simulink model "VIPLTrgtPosChk"  (R2018b)
settings: Solver=FixedStepDiscrete  StartTime=0.0  StopTime=10.0  FixedStep=0.01  RelTol=1e-3
undefined symbols (not defined in the file or in its folder): SecRwLtStBkReclnTrgtPos, SecRwLtStFwdBkwdTrgtPos, SecRwLtStLgrstInwdOtwdTrgtPos, SecRwLtStLgrstUpwdDnwdTrgtPos, SecRwLtStZeroTrgtPos, VIPL557TrgtPos_Set
settings Model: Creator=sn2xws  LastModifiedBy=sn2xws
settings Model: ModifiedHistory=|
  | 2024.7.1 V3.0.0 557模式流程V1.9
  | 2024.8.15 V3.0.1增加 avl=1反馈，avl=0时将目标位置设为最大
  | 2024.9.18 V3.0.2 智享6s，7s接口变更
  | 2024.11.15 V3.0.3 再无法计算出有效位置时，都给最小智享位置做为目标位置
settings DataIOCC: SaveFormat=StructureWithTime
settings OptimizationCC: DefaultParameterBehavior=Inlined  EnhancedBackFolding=on  PassReuseOutputArgsAs=Individual arguments  ZeroExternalMemoryAtStartup=off  ZeroInternalMemoryAtStartup=off  OptimizeBlockOrder=speed  DifferentSizesBufferReuse=on  OptimizationCustomize=off
settings DebuggingCC: ParameterTunabilityLossMsg=error
settings HardwareCC: ProdBitPerPointer=32  ProdBitPerSizeT=32  ProdBitPerPtrDiffT=32  ProdLargestAtomicFloat=None  ProdWordSize=32  ProdHWDeviceType=Renesas->RH850
settings SFSimCC: MATLABDynamicMemAlloc=off
settings SFSimCC: SimCustomHeaderCode=|
  | #include "qmath.h"
  | #include "MsminterfDet.h"
  | #include "wisenjoy.h"
settings SFSimCC: SimUserSources=|
  | qmath.c
  | MsminterfDet.c
  | wisenjoy.c
settings RTWCC: SystemTargetFile=autosar.tlc  GenCodeOnly=on  TemplateMakefile=ert_default_tmf  Description=AUTOSAR  GenerateReport=on  IncludeHyperlinkInReport=on  LaunchReport=on  GenerateTraceInfo=on  GenerateTraceReport=on  GenerateTraceReportSl=on  GenerateTraceReportSf=on  GenerateTraceReportEml=on
settings CodeAppCC: ForceParamTrailComments=on  IgnoreCustomStorageClasses=off  OperatorAnnotations=on  SimulinkDataObjDesc=on  SFDataObjDesc=on  InsertBlockDesc=on
settings STFCustomTargetCC: TargetLangStandard=C99 (ISO)  MultiwordLength=256  ParMdlRefBuildCompliant=on  CompOptLevelCompliant=on  IncludeMdlTerminateFcn=off  CombineOutputUpdateFcns=on  SuppressErrorStatus=on  ERTCustomFileBanners=on  SupportNonFinite=off  SupportComplex=off  SupportContinuousTime=off  SupportNonInlinedSFcns=off  RemoveResetFunc=on  MATLABClassNameForMDSCustomization=Simulink.SoftwareTarget.ERTCustomization  AutosarCompliant=on  UseToolchainInfoCompliant=on  LookupTableObjectStructAxisOrder=2,1,3,4,...  LUTObjectStructOrderEvenSpacing=Size,Table,Breakpoints  SystemTargetFile=autosar.tlc
settings ERTTargetCC: TargetLangStandard=C99 (ISO)  ConcurrentExecutionCompliant=off  IncludeMdlTerminateFcn=off  SuppressErrorStatus=on  SupportNonFinite=off  SupportComplex=off  ModelStepFunctionPrototypeControlCompliant=off  CPPClassGenCompliant=off  AutosarCompliant=on  LookupTableObjectStructAxisOrder=2,1,3,4,...  LUTObjectStructOrderEvenSpacing=Size,Table,Breakpoints  InlinedParameterPlacement=NonHierarchical  ERTCustomFileTemplate=example_file_process.tlc  ERTFilePackagingFormat=Compact

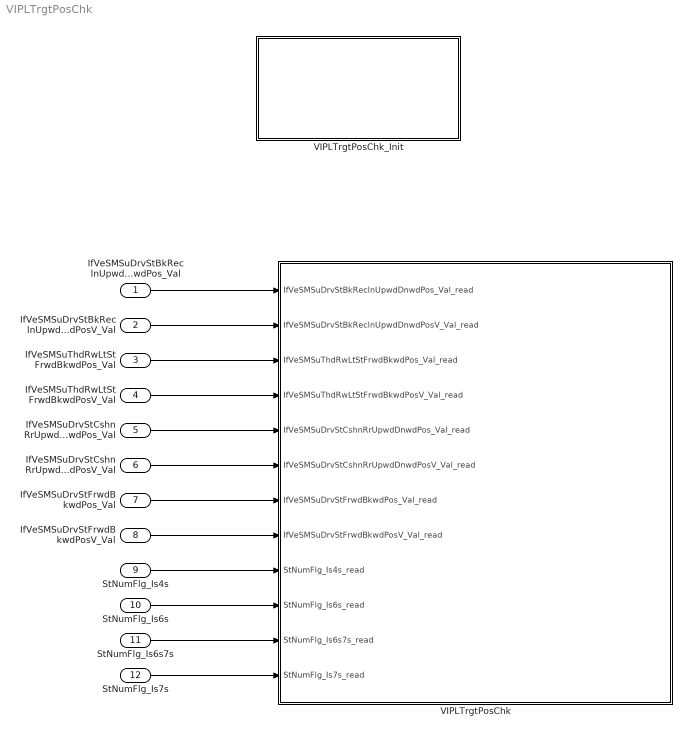
== system VIPLTrgtPosChk ==
  IfVeSMSuDrvStBkReclnUpwdDnwdPos_Val : Inport  OutDataTypeStr=uint16  PortDimensions=1
  IfVeSMSuDrvStBkReclnUpwdDnwdPosV_Val : Inport  Port=2  OutDataTypeStr=boolean  PortDimensions=1
  IfVeSMSuThdRwLtStFrwdBkwdPos_Val : Inport  Port=3  OutDataTypeStr=uint16  PortDimensions=1
  IfVeSMSuThdRwLtStFrwdBkwdPosV_Val : Inport  Port=4  OutDataTypeStr=boolean  PortDimensions=1
  IfVeSMSuDrvStCshnRrUpwdDnwdPos_Val : Inport  Port=5  OutDataTypeStr=uint16  PortDimensions=1
  IfVeSMSuDrvStCshnRrUpwdDnwdPosV_Val : Inport  Port=6  OutDataTypeStr=boolean  PortDimensions=1
  IfVeSMSuDrvStFrwdBkwdPos_Val : Inport  Port=7  OutDataTypeStr=uint16  PortDimensions=1
  IfVeSMSuDrvStFrwdBkwdPosV_Val : Inport  Port=8  OutDataTypeStr=boolean  PortDimensions=1
  StNumFlg_Is4s : Inport  Port=9  OutDataTypeStr=boolean  PortDimensions=1
  StNumFlg_Is6s : Inport  Port=10  OutDataTypeStr=boolean  PortDimensions=1
  StNumFlg_Is6s7s : Inport  Port=11  OutDataTypeStr=boolean  PortDimensions=1
  StNumFlg_Is7s : Inport  Port=12  OutDataTypeStr=boolean  PortDimensions=1
  VIPLTrgtPosChk : Subsystem
  VIPLTrgtPosChk_Init : Subsystem
  wires:
  IfVeSMSuDrvStBkReclnUpwdDnwdPos_Val/1 -> VIPLTrgtPosChk/1(IfVeSMSuDrvStBkReclnUpwdDnwdPos_Val_read)
  IfVeSMSuDrvStBkReclnUpwdDnwdPosV_Val/1 -> VIPLTrgtPosChk/2(IfVeSMSuDrvStBkReclnUpwdDnwdPosV_Val_read)
  IfVeSMSuThdRwLtStFrwdBkwdPos_Val/1 -> VIPLTrgtPosChk/3(IfVeSMSuThdRwLtStFrwdBkwdPos_Val_read)
  IfVeSMSuThdRwLtStFrwdBkwdPosV_Val/1 -> VIPLTrgtPosChk/4(IfVeSMSuThdRwLtStFrwdBkwdPosV_Val_read)
  IfVeSMSuDrvStCshnRrUpwdDnwdPos_Val/1 -> VIPLTrgtPosChk/5(IfVeSMSuDrvStCshnRrUpwdDnwdPos_Val_read)
  IfVeSMSuDrvStCshnRrUpwdDnwdPosV_Val/1 -> VIPLTrgtPosChk/6(IfVeSMSuDrvStCshnRrUpwdDnwdPosV_Val_read)
  IfVeSMSuDrvStFrwdBkwdPos_Val/1 -> VIPLTrgtPosChk/7(IfVeSMSuDrvStFrwdBkwdPos_Val_read)
  IfVeSMSuDrvStFrwdBkwdPosV_Val/1 -> VIPLTrgtPosChk/8(IfVeSMSuDrvStFrwdBkwdPosV_Val_read)
  StNumFlg_Is4s/1 -> VIPLTrgtPosChk/9(StNumFlg_Is4s_read)
  StNumFlg_Is6s/1 -> VIPLTrgtPosChk/10(StNumFlg_Is6s_read)
  StNumFlg_Is6s7s/1 -> VIPLTrgtPosChk/11(StNumFlg_Is6s7s_read)
  StNumFlg_Is7s/1 -> VIPLTrgtPosChk/12(StNumFlg_Is7s_read)

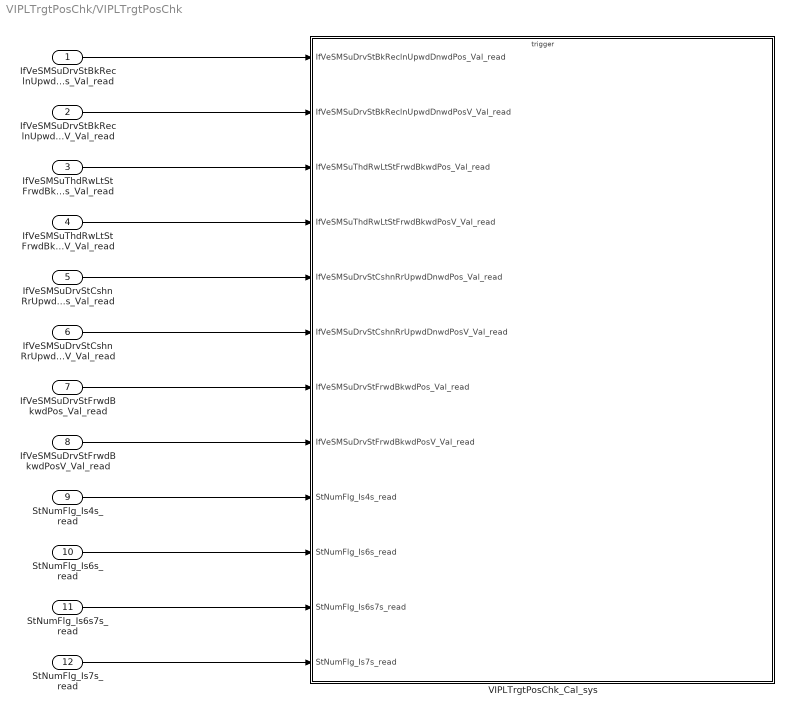
== system VIPLTrgtPosChk/VIPLTrgtPosChk ==
  IfVeSMSuDrvStBkReclnUpwdDnwdPos_Val_read : Inport
  IfVeSMSuDrvStBkReclnUpwdDnwdPosV_Val_read : Inport  Port=2
  IfVeSMSuThdRwLtStFrwdBkwdPos_Val_read : Inport  Port=3
  IfVeSMSuThdRwLtStFrwdBkwdPosV_Val_read : Inport  Port=4
  IfVeSMSuDrvStCshnRrUpwdDnwdPos_Val_read : Inport  Port=5
  IfVeSMSuDrvStCshnRrUpwdDnwdPosV_Val_read : Inport  Port=6
  IfVeSMSuDrvStFrwdBkwdPos_Val_read : Inport  Port=7
  IfVeSMSuDrvStFrwdBkwdPosV_Val_read : Inport  Port=8
  StNumFlg_Is4s_read : Inport  Port=9
  StNumFlg_Is6s_read : Inport  Port=10
  StNumFlg_Is6s7s_read : Inport  Port=11
  StNumFlg_Is7s_read : Inport  Port=12
  VIPLTrgtPosChk_Cal_sys : Subsystem
  wires:
  IfVeSMSuThdRwLtStFrwdBkwdPos_Val_read/1 -> VIPLTrgtPosChk_Cal_sys/3(IfVeSMSuThdRwLtStFrwdBkwdPos_Val_read)
  IfVeSMSuDrvStBkReclnUpwdDnwdPosV_Val_read/1 -> VIPLTrgtPosChk_Cal_sys/2(IfVeSMSuDrvStBkReclnUpwdDnwdPosV_Val_read)
  IfVeSMSuThdRwLtStFrwdBkwdPosV_Val_read/1 -> VIPLTrgtPosChk_Cal_sys/4(IfVeSMSuThdRwLtStFrwdBkwdPosV_Val_read)
  IfVeSMSuDrvStBkReclnUpwdDnwdPos_Val_read/1 -> VIPLTrgtPosChk_Cal_sys/1(IfVeSMSuDrvStBkReclnUpwdDnwdPos_Val_read)
  IfVeSMSuDrvStFrwdBkwdPosV_Val_read/1 -> VIPLTrgtPosChk_Cal_sys/8(IfVeSMSuDrvStFrwdBkwdPosV_Val_read)
  IfVeSMSuDrvStFrwdBkwdPos_Val_read/1 -> VIPLTrgtPosChk_Cal_sys/7(IfVeSMSuDrvStFrwdBkwdPos_Val_read)
  IfVeSMSuDrvStCshnRrUpwdDnwdPosV_Val_read/1 -> VIPLTrgtPosChk_Cal_sys/6(IfVeSMSuDrvStCshnRrUpwdDnwdPosV_Val_read)
  IfVeSMSuDrvStCshnRrUpwdDnwdPos_Val_read/1 -> VIPLTrgtPosChk_Cal_sys/5(IfVeSMSuDrvStCshnRrUpwdDnwdPos_Val_read)
  StNumFlg_Is4s_read/1 -> VIPLTrgtPosChk_Cal_sys/9(StNumFlg_Is4s_read)
  StNumFlg_Is6s_read/1 -> VIPLTrgtPosChk_Cal_sys/10(StNumFlg_Is6s_read)
  StNumFlg_Is6s7s_read/1 -> VIPLTrgtPosChk_Cal_sys/11(StNumFlg_Is6s7s_read)
  StNumFlg_Is7s_read/1 -> VIPLTrgtPosChk_Cal_sys/12(StNumFlg_Is7s_read)

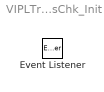
== system VIPLTrgtPosChk/VIPLTrgtPosChk_Init ==
  Event Listener : EventListener  EventName=reset

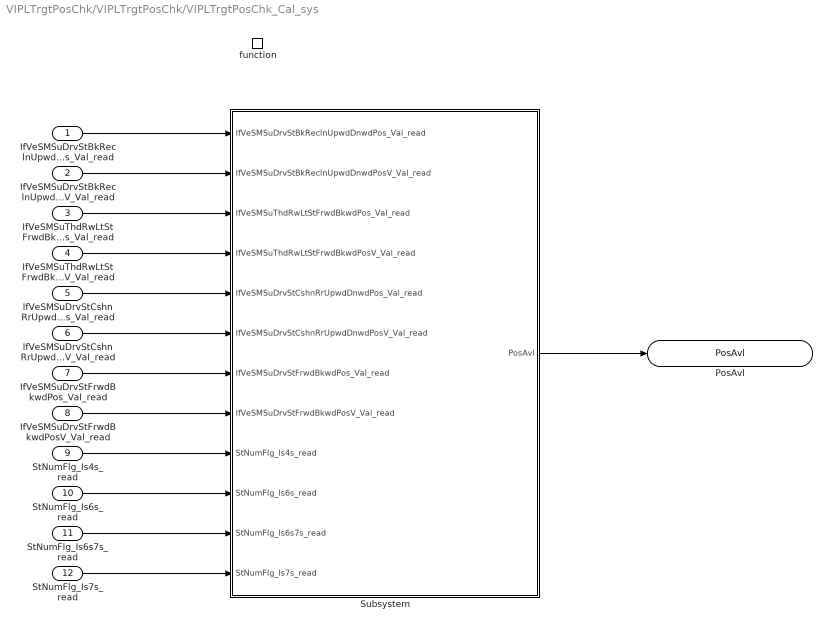
== system VIPLTrgtPosChk/VIPLTrgtPosChk/VIPLTrgtPosChk_Cal_sys ==
  IfVeSMSuDrvStBkReclnUpwdDnwdPos_Val_read : Inport
  IfVeSMSuDrvStBkReclnUpwdDnwdPosV_Val_read : Inport  Port=2
  IfVeSMSuThdRwLtStFrwdBkwdPos_Val_read : Inport  Port=3
  IfVeSMSuThdRwLtStFrwdBkwdPosV_Val_read : Inport  Port=4
  IfVeSMSuDrvStCshnRrUpwdDnwdPos_Val_read : Inport  Port=5
  IfVeSMSuDrvStCshnRrUpwdDnwdPosV_Val_read : Inport  Port=6
  IfVeSMSuDrvStFrwdBkwdPos_Val_read : Inport  Port=7
  IfVeSMSuDrvStFrwdBkwdPosV_Val_read : Inport  Port=8
  StNumFlg_Is4s_read : Inport  Port=9
  StNumFlg_Is6s_read : Inport  Port=10
  StNumFlg_Is6s7s_read : Inport  Port=11
  StNumFlg_Is7s_read : Inport  Port=12
  function : TriggerPort  TriggerType=function-call  IsSimulinkFunction=on  FunctionName=VIPLTrgtPosChk_Cal  VariantControl=(inherit)
  Subsystem : Subsystem
  PosAvl : ArgOut  OutDataTypeStr=uint8  ArgumentName=PosAvl
  wires:
  Subsystem/1(PosAvl) -> PosAvl/1
  IfVeSMSuThdRwLtStFrwdBkwdPosV_Val_read/1 -> Subsystem/4(IfVeSMSuThdRwLtStFrwdBkwdPosV_Val_read)
  IfVeSMSuDrvStBkReclnUpwdDnwdPosV_Val_read/1 -> Subsystem/2(IfVeSMSuDrvStBkReclnUpwdDnwdPosV_Val_read)
  IfVeSMSuDrvStBkReclnUpwdDnwdPos_Val_read/1 -> Subsystem/1(IfVeSMSuDrvStBkReclnUpwdDnwdPos_Val_read)
  IfVeSMSuThdRwLtStFrwdBkwdPos_Val_read/1 -> Subsystem/3(IfVeSMSuThdRwLtStFrwdBkwdPos_Val_read)
  IfVeSMSuDrvStFrwdBkwdPosV_Val_read/1 -> Subsystem/8(IfVeSMSuDrvStFrwdBkwdPosV_Val_read)
  IfVeSMSuDrvStCshnRrUpwdDnwdPos_Val_read/1 -> Subsystem/5(IfVeSMSuDrvStCshnRrUpwdDnwdPos_Val_read)
  IfVeSMSuDrvStCshnRrUpwdDnwdPosV_Val_read/1 -> Subsystem/6(IfVeSMSuDrvStCshnRrUpwdDnwdPosV_Val_read)
  IfVeSMSuDrvStFrwdBkwdPos_Val_read/1 -> Subsystem/7(IfVeSMSuDrvStFrwdBkwdPos_Val_read)
  StNumFlg_Is6s7s_read/1 -> Subsystem/11(StNumFlg_Is6s7s_read)
  StNumFlg_Is7s_read/1 -> Subsystem/12(StNumFlg_Is7s_read)
  StNumFlg_Is4s_read/1 -> Subsystem/9(StNumFlg_Is4s_read)
  StNumFlg_Is6s_read/1 -> Subsystem/10(StNumFlg_Is6s_read)

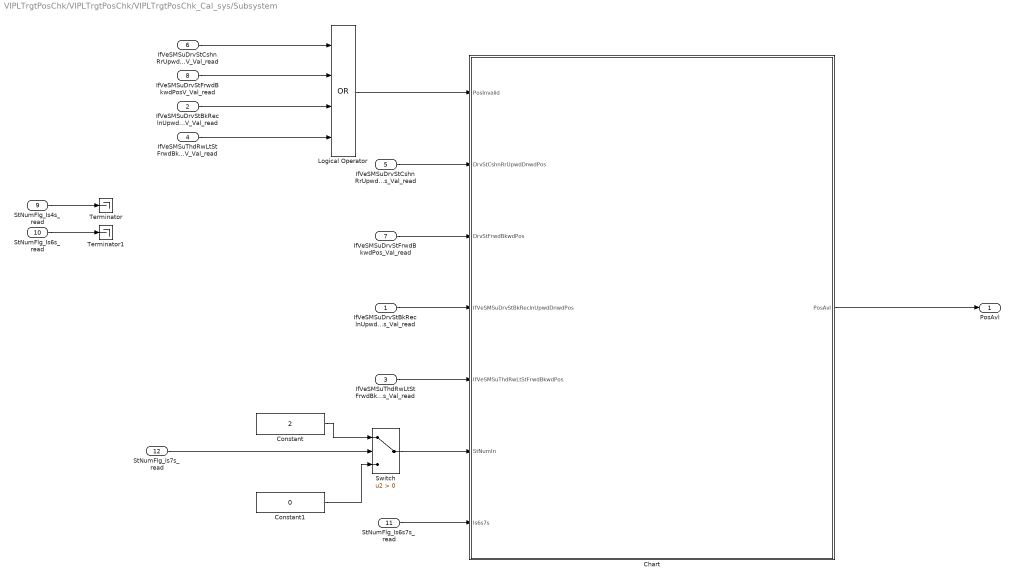
== system VIPLTrgtPosChk/VIPLTrgtPosChk/VIPLTrgtPosChk_Cal_sys/Subsystem ==
  IfVeSMSuDrvStBkReclnUpwdDnwdPos_Val_read : Inport
  IfVeSMSuDrvStBkReclnUpwdDnwdPosV_Val_read : Inport  Port=2
  IfVeSMSuThdRwLtStFrwdBkwdPos_Val_read : Inport  Port=3
  IfVeSMSuThdRwLtStFrwdBkwdPosV_Val_read : Inport  Port=4
  IfVeSMSuDrvStCshnRrUpwdDnwdPos_Val_read : Inport  Port=5
  IfVeSMSuDrvStCshnRrUpwdDnwdPosV_Val_read : Inport  Port=6
  IfVeSMSuDrvStFrwdBkwdPos_Val_read : Inport  Port=7
  IfVeSMSuDrvStFrwdBkwdPosV_Val_read : Inport  Port=8
  StNumFlg_Is4s_read : Inport  Port=9
  StNumFlg_Is6s_read : Inport  Port=10
  StNumFlg_Is6s7s_read : Inport  Port=11
  StNumFlg_Is7s_read : Inport  Port=12
  Chart : Stateflow chart  TreatAsAtomicUnit=on
  Constant : Constant  Value=2  OutDataTypeStr=uint8
  Constant1 : Constant  Value=0  OutDataTypeStr=uint8
  Logical Operator : Logic  Operator=OR  Inputs=4  AllPortsSameDT=off  OutDataTypeStr=boolean
  Switch : Switch  Criteria=u2 > Threshold
  Terminator : Terminator
  Terminator1 : Terminator
  PosAvl : Outport
  wires:
  Chart/1(PosAvl) -> PosAvl/1
  IfVeSMSuThdRwLtStFrwdBkwdPosV_Val_read/1 -> Logical Operator/4
  IfVeSMSuDrvStBkReclnUpwdDnwdPosV_Val_read/1 -> Logical Operator/3
  IfVeSMSuDrvStBkReclnUpwdDnwdPos_Val_read/1 -> Chart/4(IfVeSMSuDrvStBkReclnUpwdDnwdPos)
  IfVeSMSuThdRwLtStFrwdBkwdPos_Val_read/1 -> Chart/5(IfVeSMSuThdRwLtStFrwdBkwdPos)
  Logical Operator/1 -> Chart/1(PosInvalid)
  IfVeSMSuDrvStCshnRrUpwdDnwdPos_Val_read/1 -> Chart/2(DrvStCshnRrUpwdDnwdPos)
  IfVeSMSuDrvStFrwdBkwdPos_Val_read/1 -> Chart/3(DrvStFrwdBkwdPos)
  IfVeSMSuDrvStCshnRrUpwdDnwdPosV_Val_read/1 -> Logical Operator/1
  IfVeSMSuDrvStFrwdBkwdPosV_Val_read/1 -> Logical Operator/2
  StNumFlg_Is4s_read/1 -> Terminator/1
  StNumFlg_Is6s_read/1 -> Terminator1/1
  StNumFlg_Is7s_read/1 -> Switch/2
  Constant/1 -> Switch/1
  Constant1/1 -> Switch/3
  Switch/1 -> Chart/6(StNumIn)
  StNumFlg_Is6s7s_read/1 -> Chart/7(Is6s7s)

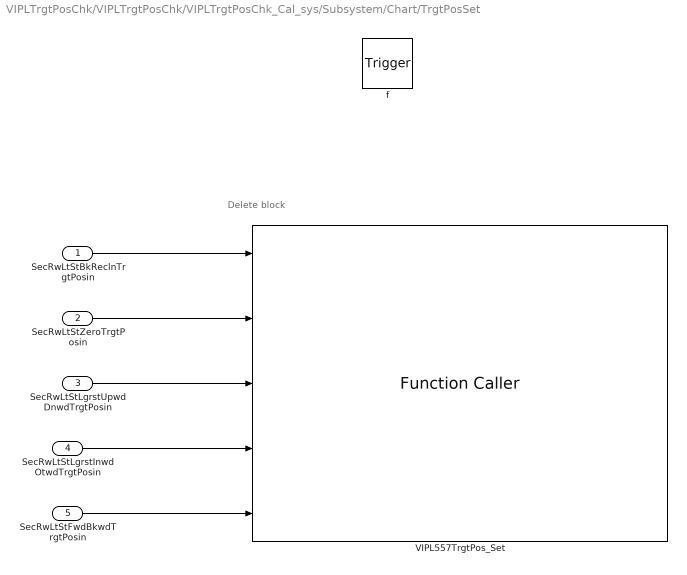
== system VIPLTrgtPosChk/VIPLTrgtPosChk/VIPLTrgtPosChk_Cal_sys/Subsystem/Chart/TrgtPosSet ==
  note: Delete block
  SecRwLtStBkReclnTrgtPosin : Inport
  SecRwLtStZeroTrgtPosin : Inport  Port=2
  SecRwLtStLgrstUpwdDnwdTrgtPosin : Inport  Port=3
  SecRwLtStLgrstInwdOtwdTrgtPosin : Inport  Port=4
  SecRwLtStFwdBkwdTrgtPosin : Inport  Port=5
  f : TriggerPort  TriggerType=function-call  VariantControl=(inherit)
      settings: CopyFcn=Stateflow.SLINSF.SimulinkMan.removeBlockPreDeleteFcn  PreDeleteFcn=Stateflow.SLINSF.SimulinkMan.unsafePredeleteFcn
  VIPL557TrgtPos_Set : FunctionCaller  FunctionPrototype=VIPL557TrgtPos_Set(SecRwLtStBkReclnTrgtPos,SecRwLtStZeroTrgtPos,SecRwLtStLgrstUpwdDnwdTrgtPos,SecRwLtStLgrstInwdOtwdTrgtPos,SecRwLtStFwdBkwdTrgtPos)  InputArgumentSpecifications=uint16(1), uint16(1), uint16(1), uint16(1), uint16(1)
  wires:
  SecRwLtStBkReclnTrgtPosin/1 -> VIPL557TrgtPos_Set/1
  SecRwLtStZeroTrgtPosin/1 -> VIPL557TrgtPos_Set/2
  SecRwLtStLgrstUpwdDnwdTrgtPosin/1 -> VIPL557TrgtPos_Set/3
  SecRwLtStLgrstInwdOtwdTrgtPosin/1 -> VIPL557TrgtPos_Set/4
  SecRwLtStFwdBkwdTrgtPosin/1 -> VIPL557TrgtPos_Set/5

== stateflow chart VIPLTrgtPosChk/VIPLTrgtPosChk_Cal_sys/Subsystem/Chart ==
  state TrgtPosSet(SecRwLtStBkReclnTrgtPosin,SecRwLtStZeroTrgtPosin,SecRwLtStLgrstUpwdDnwdTrgtPosin,SecRwLtStLgrstInwdOtwdTrgtPosin,SecRwLtStFwdBkwdTrgtPosin) [function]
  (default) -> (junction 2)
  (junction 2) -> (junction 6) [order 1] : [PosInvalid||!Is6s7s]
  (junction 2) -> (junction 53) [order 2] : {
      | r1mhin = DrvStCshnRrUpwdDnwdPos;
      | r1mhin = r1mhin/4000;
      | r1mfin = DrvStFrwdBkwdPos;
      | r1mfin = r1mfin/4000;
      | r1mbin = IfVeSMSuDrvStBkReclnUpwdDnwdPos;
      | r1mbin = r1mbin/4000;
      | r3mfin = IfVeSMSuThdRwLtStFrwdBkwdPos;
      | r3mfin = r3mfin/4000;
      | }
  (junction 6) -> (junction 158)
  (junction 53) -> (junction 158) [order 1] : [MsmInterfDet_WisdomEnjoySearch(StNumIn,r1mhin,r1mbin,r1mfin,r3mfin)<=0]
  (junction 53) -> (junction 100) [order 2] : {
      | ans = MsmInterfDet_GetAns();
      | }
  (junction 158) -> (junction 8) : {PosAvl = 1;
      | TrgtPosSet(1902,0,2400,4000,4000);
      | }
  (junction 100) -> (junction 4) : {
      | SecRwLtFwdBkwdTrgtPos = ans.ans_r2mf*4000;
      | SecRwLtStZeroTrgtPos = ans.ans_r2m0*4000;
      | SecRwLtStBkReclnTrgtPos =ans.ans_r2mb*4000;
      | SecRwLtStLgrstUpwdDnwdTrgtPos = ans.ans_r2ml*4000;
      | %SecRwLtStLgrstInwdOtwdTrgtPos =ans.ans_r2me*4000;
      | SecRwLtStLgrstInwdOtwdTrgtPos = 4000;
      | TrgtPosSet(SecRwLtStBkReclnTrgtPos,SecRwLtStZeroTrgtPos,SecRwLtStLgrstUpwdDnwdTrgtPos,SecRwLtStLgrstInwdOtwdTrgtPos,SecRwLtFwdBkwdTrgtPos);
      | PosAvl =1;
      | }
  (junction 8) -> (junction 4)
  (junction 4) -> (junction 96)
  data: SecRwLtStBkReclnTrgtPosin function_input; SecRwLtStZeroTrgtPosin function_input; SecRwLtStLgrstUpwdDnwdTrgtPosin function_input; SecRwLtStLgrstInwdOtwdTrgtPosin function_input; SecRwLtStFwdBkwdTrgtPosin function_input; PosAvl output; SecRwLtStBkReclnTrgtPos local uint16; SecRwLtStZeroTrgtPos local uint16; SecRwLtStLgrstUpwdDnwdTrgtPos local uint16; SecRwLtStLgrstInwdOtwdTrgtPos local uint16; SecRwLtFwdBkwdTrgtPos local uint16; PosInvalid input boolean; DrvStCshnRrUpwdDnwdPos input uint16; DrvStFrwdBkwdPos input uint16; IfVeSMSuDrvStBkReclnUpwdDnwdPos input uint16; IfVeSMSuThdRwLtStFrwdBkwdPos input uint16; r1mhin local single; r1mbin local single; r1mfin local single; r3mfin local single; ans local Bus: MsmAnsTyp; StNumIn input uint8; Is6s7s input boolean
